simulink model "untitled"  (R2023a)
settings: Solver=VariableStepAuto  StartTime=0.0  StopTime=1  RelTol=1e-3
settings Model: Creator=VICTOR7  LastModifiedBy=VICTOR7

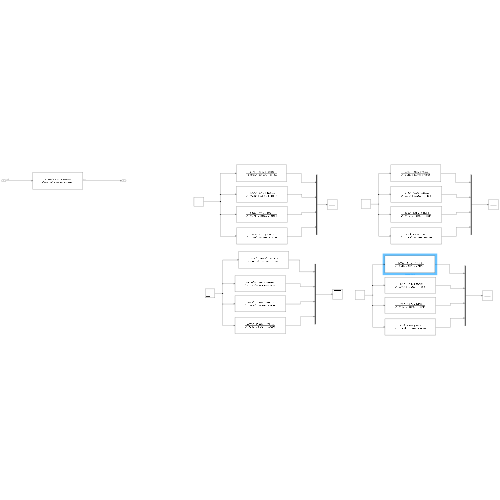
[thumbnail: Simulink's stored preview of the top-level diagram]
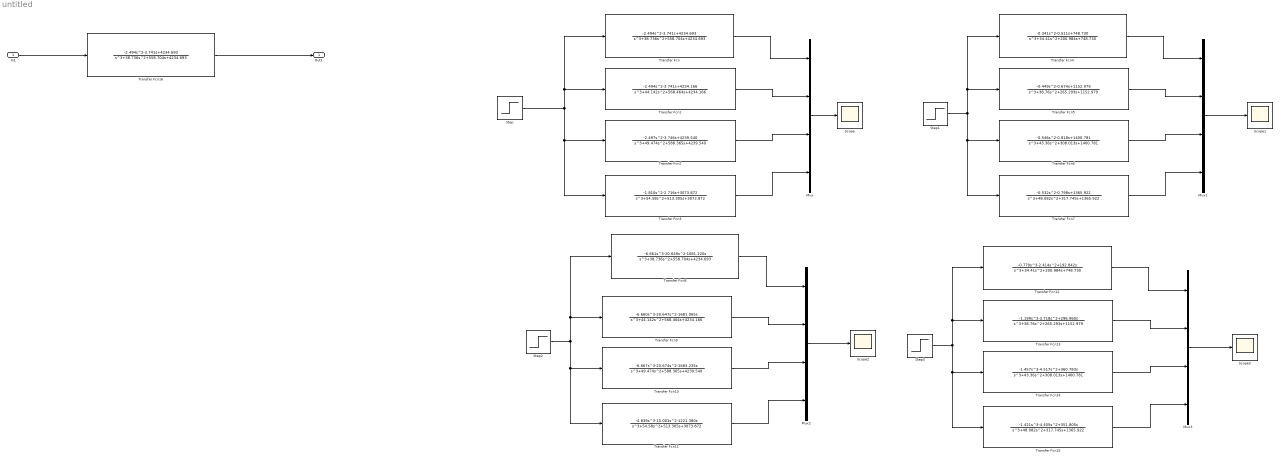
== system untitled ==
  In1 : Inport
  Mux{,1..3} (4 alike) : Mux
  Scope{,1..3} (4 alike) : Scope
  Step{,1..3} (4 alike) : Step  Time=0  SampleTime=0
  Transfer Fcn : TransferFcn  Numerator=[-2.494 -3.741 4234.693]  Denominator=[1 38.736 558.704 4234.693]
  Transfer Fcn1 : TransferFcn  Numerator=[-2.494 -3.741 4234.166]  Denominator=[1 44.142 568.464 4234.166]
  Transfer Fcn10 : TransferFcn  Numerator=[-6.667 -20.674 -1683.235 0]  Denominator=[1 49.474 588.365 4239.540]
  Transfer Fcn11 : TransferFcn  Numerator=[-4.839 -15.001 -1221.380 0]  Denominator=[1 54.58 513.305 3073.872]
  Transfer Fcn12 : TransferFcn  Numerator=[-0.779 -2.414 192.842 0]  Denominator=[1 34.41 200.984 748.730]
  Transfer Fcn13 : TransferFcn  Numerator=[-1.199 -3.718 296.960 0]  Denominator=[1 38.76 265.293 1152.979]
  Transfer Fcn14 : TransferFcn  Numerator=[-1.457 -4.517 360.783 0]  Denominator=[1 43.36 308.013 1400.781]
  Transfer Fcn15 : TransferFcn  Numerator=[-1.421 -4.405 351.805 0]  Denominator=[1 48.082 317.745 1365.922]
  Transfer Fcn16 : TransferFcn  Numerator=[-2.494 -3.741 4234.693]  Denominator=[1 38.736 558.704 4234.693]
  Transfer Fcn2 : TransferFcn  Numerator=[-2.497 -3.746 4239.540]  Denominator=[1 49.474 588.365 4239.540]
  Transfer Fcn3 : TransferFcn  Numerator=[-1.810 -2.716 3073.872]  Denominator=[1 54.58 513.305 3073.872]
  Transfer Fcn4 : TransferFcn  Numerator=[-0.341 -0.511 748.730]  Denominator=[1 34.41 200.984 748.730]
  Transfer Fcn5 : TransferFcn  Numerator=[-0.449 -0.674 1152.979]  Denominator=[1 38.76 265.293 1152.979]
  Transfer Fcn6 : TransferFcn  Numerator=[-0.546 -0.818 1400.781]  Denominator=[1 43.36 308.013 1400.781]
  Transfer Fcn7 : TransferFcn  Numerator=[-0.532 -0.798 1365.922]  Denominator=[1 48.082 317.745 1365.922]
  Transfer Fcn8 : TransferFcn  Numerator=[-6.661 -20.649 -1681.220 0]  Denominator=[1 38.736 558.704 4234.693]
  Transfer Fcn9 : TransferFcn  Numerator=[-6.660 -20.647 -1681.065 0]  Denominator=[1 44.142 568.464 4234.166]
  Out1 : Outport
  wires:
  Transfer Fcn/1 -> Mux/1
  Transfer Fcn1/1 -> Mux/2
  Transfer Fcn2/1 -> Mux/3
  Transfer Fcn3/1 -> Mux/4
  Transfer Fcn4/1 -> Mux1/1
  Transfer Fcn7/1 -> Mux1/4
  Mux1/1 -> Scope1/1
  Step1/1 -> Transfer Fcn4/1, Transfer Fcn5/1, Transfer Fcn7/1, Transfer Fcn6/1
  Transfer Fcn6/1 -> Mux1/3
  Transfer Fcn5/1 -> Mux1/2
  Transfer Fcn8/1 -> Mux2/1
  Transfer Fcn11/1 -> Mux2/4
  Mux2/1 -> Scope2/1
  Step2/1 -> Transfer Fcn8/1, Transfer Fcn9/1, Transfer Fcn11/1, Transfer Fcn10/1
  Transfer Fcn10/1 -> Mux2/3
  Transfer Fcn9/1 -> Mux2/2
  Step3/1 -> Transfer Fcn12/1, Transfer Fcn13/1, Transfer Fcn15/1, Transfer Fcn14/1
  Mux3/1 -> Scope3/1
  Transfer Fcn12/1 -> Mux3/1
  Transfer Fcn15/1 -> Mux3/4
  Transfer Fcn14/1 -> Mux3/3
  Transfer Fcn13/1 -> Mux3/2
  Step/1 -> Transfer Fcn/1, Transfer Fcn1/1, Transfer Fcn3/1, Transfer Fcn2/1
  Mux/1 -> Scope/1
  Transfer Fcn16/1 -> Out1/1
  In1/1 -> Transfer Fcn16/1
